simulink model "simulation_system"  (R2019a)
settings: Solver=VariableStepAuto  StartTime=0.0  StopTime=720000  RelTol=1e-3
settings Model: Creator=86180  LastModifiedBy=86180
settings OptimizationCC: DefaultParameterBehavior=Inlined  EnhancedBackFolding=on  PassReuseOutputArgsAs=Individual arguments  OptimizeBlockOrder=speed  DifferentSizesBufferReuse=on  OptimizationCustomize=off
settings DebuggingCC: ParameterTunabilityLossMsg=error
settings SFSimCC: MATLABDynamicMemAlloc=off
settings RTWCC: SystemTargetFile=ert.tlc  GenCodeOnly=on  PackageGeneratedCodeAndArtifacts=on  PackageName=sumulation_system  TemplateMakefile=ert_default_tmf  GenerateReport=on  IncludeHyperlinkInReport=on  LaunchReport=on  GenerateTraceInfo=on  GenerateTraceReport=on  GenerateTraceReportSl=on  GenerateTraceReportSf=on  GenerateTraceReportEml=on
settings CodeAppCC: ForceParamTrailComments=on  IgnoreCustomStorageClasses=off  OperatorAnnotations=on  SimulinkDataObjDesc=on  SFDataObjDesc=on  InsertBlockDesc=on
settings ERTTargetCC: TargetLangStandard=C99 (ISO)  GenerateSampleERTMain=on  InlinedParameterPlacement=NonHierarchical  ERTCustomFileTemplate=example_file_process.tlc

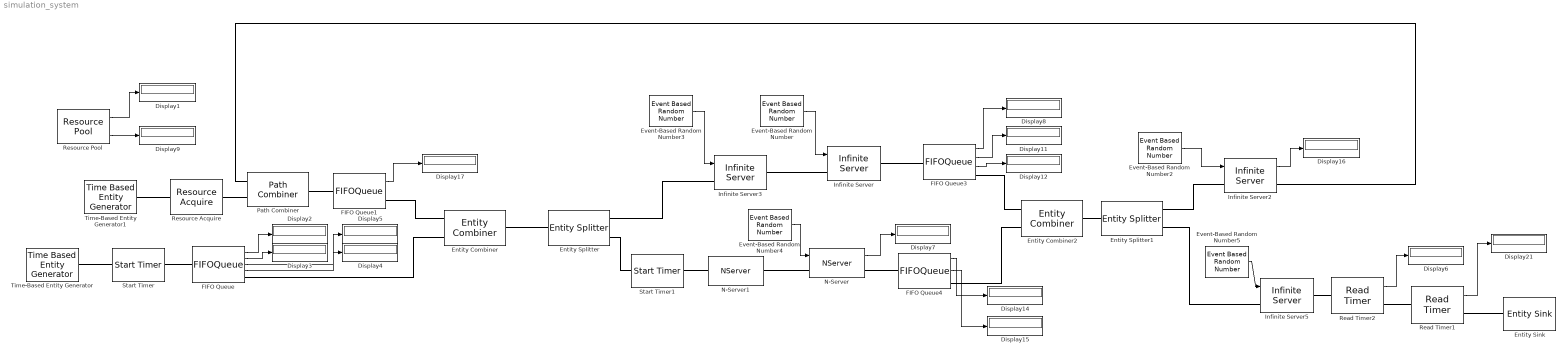
== system simulation_system ==
  Display{1..9,11..12,14..17,21} (16 alike) : Display
  Entity Combiner : EntityCombiner  NumberInputPorts=2
  Entity Combiner2 : EntityCombiner  NumberInputPorts=2
  Entity Sink : EntitySink
  Entity Splitter : EntitySplitter  NumberOutputPorts=2
  Entity Splitter1 : EntitySplitter  NumberOutputPorts=2
  Event-Based Random Number : EventBasedRandomNumber  meanExp=387  meanNorm=315  stdNorm=5  Seed=34425
  Event-Based Random Number2 : EventBasedRandomNumber  meanExp=10  Seed=58140
  Event-Based Random Number3 : EventBasedRandomNumber  meanExp=10  meanNorm=12  stdNorm=3  Seed=11223
  Event-Based Random Number4 : EventBasedRandomNumber  meanExp=986  meanNorm=7  stdNorm=38  Seed=343
  Event-Based Random Number5 : EventBasedRandomNumber  meanExp=10  Seed=61357
  FIFO Queue : FIFOQueue  Capacity=10000  StatNumberDeparted=on  StatNumberInBlock=on  StatAverageWait=on  StatAverageQueueLength=on
      settings: OutputPortMap=o0,o1,o2,o3
  FIFO Queue1 : FIFOQueue  StatAverageQueueLength=on
      settings: OutputPortMap=o3
  FIFO Queue3 : FIFOQueue  StatNumberDeparted=on  StatAverageWait=on  StatAverageQueueLength=on
      settings: OutputPortMap=o0,o2,o3
  FIFO Queue4 : FIFOQueue  Capacity=1  StatAverageWait=on  StatAverageQueueLength=on
      settings: OutputPortMap=o2,o3
  Infinite Server : InfiniteServer  ServiceTimeFrom=Signal port t
  Infinite Server2 : InfiniteServer  ServiceTimeFrom=Signal port t  StatNumberDeparted=on
  Infinite Server3 : InfiniteServer  ServiceTimeFrom=Signal port t
  Infinite Server5 : InfiniteServer  ServiceTimeFrom=Signal port t
  N-Server : NServer  NumberOfServers=48  ServiceTimeFrom=Signal port t  StatUtilization=on
      settings: OutputPortMap=o5
  N-Server1 : NServer  NumberOfServers=20  ServiceTime=0
  Path Combiner : PathCombiner  NumberInputPorts=2
  Read Timer1 : ReadTimer  TimerTag=T2  StatAverageTimeElapsed=on
      settings: OutputPortMap=o3
  Read Timer2 : ReadTimer  StatAverageTimeElapsed=on
      settings: OutputPortMap=o3
  Resource Acquire : ResourceAcquire  ResourceName=robot  Capacity=100  EvaluatedResourceAmount={ 1}
  Resource Pool : ResourcePool  ResourceName=robot  ResourceAmount=48  StatAmountInUse=on  StatUtilization=on
      settings: OutputPortMap=o0,o1
  Start Timer : StartTimer  TimerTag=T2  TimerStartedOption=Continue
  Start Timer1 : StartTimer  TimerStartedOption=Continue
  Time-Based Entity Generator : TimeBasedEntityGenerator  Distribution=Exponential  InitialSeed=40859  Mean=3600/60
  Time-Based Entity Generator1 : TimeBasedEntityGenerator  Period=0.00000001  Mean=3600/20
  wires:
  FIFO Queue/3 -> Display5/1
  Infinite Server2/1 -> Display16/1
  FIFO Queue/4 -> Display4/1
  Read Timer1/1 -> Display21/1
  FIFO Queue4/1 -> Display14/1
  FIFO Queue4/2 -> Display15/1
  FIFO Queue/1 -> Display2/1
  FIFO Queue3/3 -> Display12/1
  FIFO Queue3/1 -> Display8/1
  Event-Based Random Number2/1 -> Infinite Server2/1
  Event-Based Random Number3/1 -> Infinite Server3/1
  Event-Based Random Number/1 -> Infinite Server/1
  FIFO Queue3/2 -> Display11/1
  Resource Pool/1 -> Display1/1
  FIFO Queue/2 -> Display3/1
  Event-Based Random Number5/1 -> Infinite Server5/1
  Event-Based Random Number4/1 -> N-Server/1
  Read Timer2/1 -> Display6/1
  N-Server/1 -> Display7/1
  Resource Pool/2 -> Display9/1
  FIFO Queue1/1 -> Display17/1
  connections:
  FIFO Queue1/LConn1 -- Path Combiner/RConn1
  FIFO Queue1/RConn1 -- Entity Combiner/LConn1
  FIFO Queue4/RConn1 -- Entity Combiner2/LConn2
  Path Combiner/LConn1 -- Infinite Server2/RConn1
  Entity Splitter/RConn1 -- Infinite Server3/LConn1
  Infinite Server3/RConn1 -- Infinite Server/LConn1
  FIFO Queue3/RConn1 -- Entity Combiner2/LConn1
  Start Timer1/LConn1 -- Entity Splitter/RConn2
  Time-Based Entity Generator1/RConn1 -- Resource Acquire/LConn1
  N-Server/RConn1 -- FIFO Queue4/LConn1
  FIFO Queue/RConn1 -- Entity Combiner/LConn2
  Resource Acquire/RConn1 -- Path Combiner/LConn2
  FIFO Queue3/LConn1 -- Infinite Server/RConn1
  Entity Splitter/LConn1 -- Entity Combiner/RConn1
  Time-Based Entity Generator/RConn1 -- Start Timer/LConn1
  Entity Splitter1/LConn1 -- Entity Combiner2/RConn1
  Entity Splitter1/RConn1 -- Infinite Server2/LConn1
  Entity Splitter1/RConn2 -- Infinite Server5/LConn1
  Start Timer/RConn1 -- FIFO Queue/LConn1
  Read Timer1/RConn1 -- Entity Sink/LConn1
  Read Timer2/LConn1 -- Infinite Server5/RConn1
  Read Timer2/RConn1 -- Read Timer1/LConn1
  Start Timer1/RConn1 -- N-Server1/LConn1
  N-Server1/RConn1 -- N-Server/LConn1
